simulink model "COMA_CR1"  (R2023b)
settings: Solver=VariableStepAuto  StartTime=0.0  StopTime=150  RelTol=1e-3
InitFcn:
  | data
values from neighbouring files (symbols this model uses):
  G = 5    [data.m]
  K = 0.1118    [data.m]
  Kc = 1/18    (= 0.0555555555556)    [data.m]
  tau = 2*10^(-2)    (= 0.02)    [data.m]
settings Model: Creator=yannm  LastModifiedBy=yannm

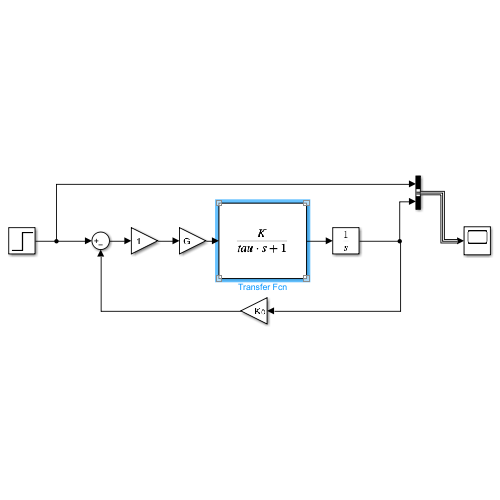
[thumbnail: Simulink's stored preview of the top-level diagram]
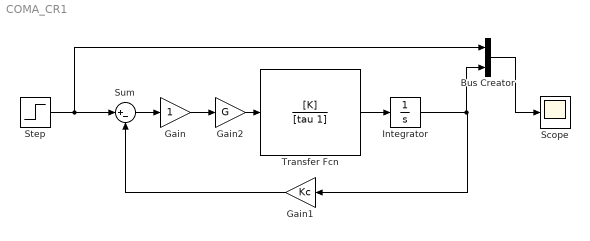
== system COMA_CR1 ==
  Bus Creator : BusCreator  Inputs=2
  Gain : Gain
  Gain1 : Gain  Gain=Kc
  Gain2 : Gain  Gain=G
  Integrator : Integrator
  Scope : Scope
  Step : Step  Time=0.5  SampleTime=0
  Sum : Sum  Inputs=|+-
  Transfer Fcn : TransferFcn  Numerator=[K]  Denominator=[tau 1]
  wires:
  Transfer Fcn/1 -> Integrator/1
  Sum/1 -> Gain/1
  Integrator/1 -> Bus Creator/2, Gain1/1
  Gain1/1 -> Sum/2
  Step/1 -> Bus Creator/1, Sum/1
  Bus Creator/1 -> Scope/1
  Gain/1 -> Gain2/1
  Gain2/1 -> Transfer Fcn/1
